simulink model "raspberrypi_I2C_temp"  (R2018b)
settings: Solver=FixedStepAuto  StartTime=0.0  StopTime=inf  RelTol=1e-3
undefined symbols (not defined in the file or in its folder): Green, led0
libraries: raspberrypilib x1, embdlinuxlib x1, realtime_examples_misc x1
settings Model: SimulationMode=external  ExtModeTrigDuration=2  Creator=The MathWorks, Inc.  LastModifiedBy=The MathWorks, Inc.
settings SolverCC: PositivePriorityOrder=on
settings DataIOCC: LimitDataPoints=on
settings OptimizationCC: BlockReduction=off  LifeSpan=Inf  MaxStackSize=64
settings DebuggingCC: AllowSymbolicDim=off  SFUnexpectedBacktrackingDiag=warning  SFNoUnconditionalDefaultTransitionDiag=warning  SFExecutionAtInitializationDiag=none
settings HardwareCC: ProdBitPerPointer=32  ProdBitPerSizeT=32  ProdBitPerPtrDiffT=32  ProdLargestAtomicInteger=Long  ProdLargestAtomicFloat=Double  ProdWordSize=32  ProdHWDeviceType=ARM Compatible->ARM Cortex  UseEmbeddedCoderFeatures=off  UseSimulinkCoderFeatures=off
settings ModelReferenceCC: PropagateSignalLabelsOutOfModel=off
settings SFSimCC: SimUseLocalCustomCode=off
settings RTWCC: SystemTargetFile=ert.tlc  HardwareBoard=Raspberry Pi  TemplateMakefile=ert_default_tmf  RTWUseLocalCustomCode=off  Toolchain=GNU GCC Raspberry Pi  BuildConfiguration=Faster Runs
settings CodeAppCC: StateflowObjectComments=on
settings ERTTargetCC: MultiwordLength=2048  ERTCustomFileBanners=off  SupportContinuousTime=on  SupportNonInlinedSFcns=on  RemoveResetFunc=off  SupportVariableSizeSignals=on  ModelStepFunctionPrototypeControlCompliant=off  ConvertIfToSwitch=off  SuppressUnreachableDefaultCases=off
settings ConfigComp: CovMetricSettings=dw  CovHtmlReporting=on  CovSaveCumulativeToWorkspaceVar=on  CovSaveSingleToWorkspaceVar=on  CovExternalEMLEnable=off

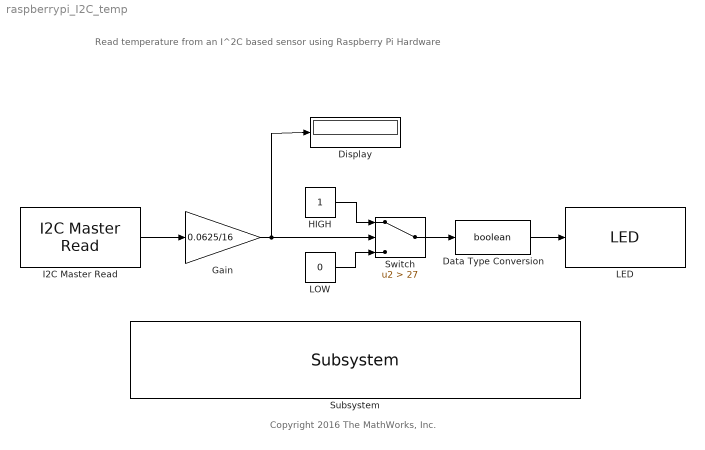
== system raspberrypi_I2C_temp ==
  note: Copyright 2016 The MathWorks, Inc.
  note: Read temperature from an I^2C based sensor
      | using Raspberry Pi Hardware
  Data Type Conversion : DataTypeConversion  OutDataTypeStr=boolean
  Display : Display
  Gain : Gain  Gain=0.0625/16  OutDataTypeStr=single
  HIGH : Constant  OutDataTypeStr=uint8
  I2C Master Read : raspberrypilib/I2C Master Read  BoardProperty=Pi 3 Model B  Mode=Master  SlaveAddress=hex2dec('48')  SlaveByteOrder=BigEndian  Direction=Receiver  RegisterAddressMode=off  RegisterAddress=0  SlaveDataType=int16  DataLength=1  NoAck=off  RepeatedStart=off  OutputStatus=off  SampleTime=0.1
      settings: SourceProductName=Simulink Support Package for Raspberry Pi Hardware  SourceProductBaseCode=RASPPI
  LED : embdlinuxlib/LED  board=Model B+  led=led0 (Green)  blockPlatform=Raspberry Pi
      settings: SourceProductName=Simulink Support Package for Raspberry Pi Hardware  SourceProductBaseCode=RASPPI
  LOW : Constant  Value=0  OutDataTypeStr=uint8
  Subsystem : realtime_examples_misc/Subsystem  SystemSampleTime=-1
  Switch : Switch  Criteria=u2 > Threshold  Threshold=27
  wires:
  I2C Master Read/1 -> Gain/1
  Gain/1 -> Display/1, Switch/2
  Data Type Conversion/1 -> LED/1
  Switch/1 -> Data Type Conversion/1
  HIGH/1 -> Switch/1
  LOW/1 -> Switch/3
